simulink model "rocky_motor_disturb"  (R2022a)
settings: Solver=VariableStepAuto  StartTime=0.0  StopTime=2  RelTol=1e-3
model workspace (MAT data in the model file):
  m = 1000
values from neighbouring files (symbols this model uses):
  ci = 1    [rocky_constants.m]
  g = 9.81    [Rocky_closed_loop_poles.m]    (also in Rocky_closed_loop_poles_again.m; Rocky_closed_loop_poles_fresh_file.m; polederivation_CA.m; rocky_constants.m = 9.8)
  ji = 10    [rocky_constants.m]
  jp = 20    [rocky_constants.m]
  ki = 1.9509e+03    (= 1950.9)    [rocky_constants.m]
  kmotor = .92    (= 0.92)    [rocky_constants.m]
  kp = 2.2104e+03    (= 2210.4)    [rocky_constants.m]
  l = 0.4529    [Rocky_closed_loop_poles.m]    (also in Rocky_closed_loop_poles_again.m = 0.5588; Rocky_closed_loop_poles_fresh_file.m = 0.5588; polederivation_CA.m = 0.45; rocky_constants.m = 0.4)
  tau = .0511    (= 0.0511)    [rocky_constants.m]
settings Model: Creator=clee1  LastModifiedBy=ayydin
settings SolverCC: AlgebraicLoopSolver=TrustRegion
settings DebuggingCC: UnconnectedInputMsg=warning  UnconnectedOutputMsg=warning  UnconnectedLineMsg=warning  SFMachineParentedDataDiag=warning

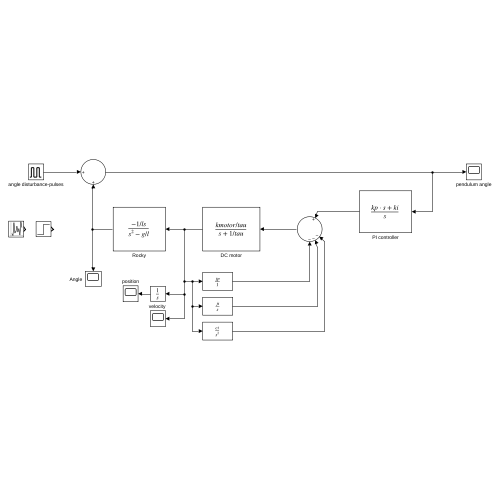
[thumbnail: Simulink's stored preview of the top-level diagram]
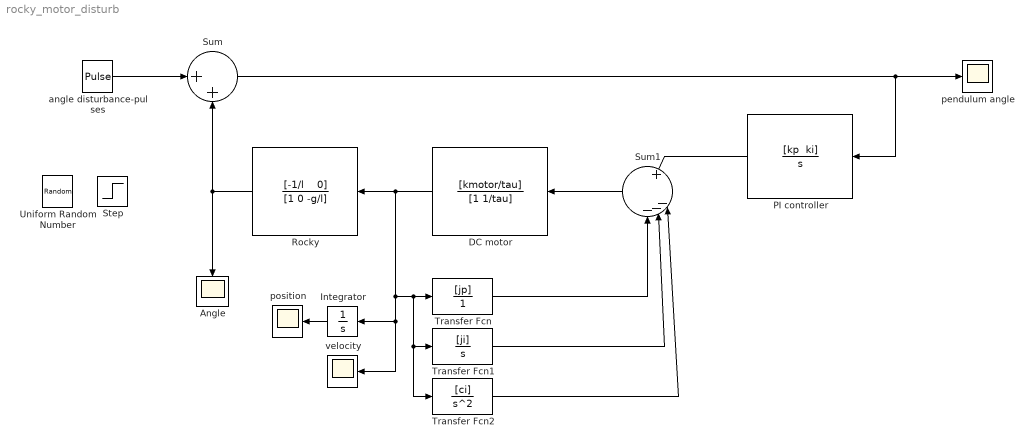
== system rocky_motor_disturb ==
  Angle : Scope
  DC motor : TransferFcn  Numerator=[kmotor/tau]  Denominator=[1 1/tau]
  Integrator : Integrator
  PI controller : TransferFcn  Numerator="[kp  ki]"  Denominator=[1 0 ]
  Rocky : TransferFcn  Numerator="[-1/l    0]"  Denominator=[1 0 -g/l]
  Step : Step  After=.1  SampleTime=0
  Sum : Sum  Inputs=|++
  Sum1 : Sum  Inputs=|+|||---
  Transfer Fcn : TransferFcn  Numerator=[jp]  Denominator=[1]
  Transfer Fcn1 : TransferFcn  Numerator=[ji]  Denominator=[1 0]
  Transfer Fcn2 : TransferFcn  Numerator=[ci]  Denominator=[1 0 0]
  Uniform Random Number : UniformRandomNumber  SampleTime=20
  angle disturbance-pulses : DiscretePulseGenerator  PulseType=Time based  Amplitude=.1  Period=10  PulseWidth=.1  PhaseDelay=.5
  pendulum angle : Scope
  position : Scope
  "velocity " : Scope
  wires:
  Rocky/1 -> Sum/2, Angle/1
  Sum/1 -> PI controller/1, pendulum angle/1
  angle disturbance-pulses/1 -> Sum/1
  DC motor/1 -> Transfer Fcn2/1, Transfer Fcn1/1, Transfer Fcn/1, "velocity "/1, Integrator/1, Rocky/1
  Integrator/1 -> position/1
  PI controller/1 -> Sum1/1
  Sum1/1 -> DC motor/1
  Transfer Fcn/1 -> Sum1/4
  Transfer Fcn1/1 -> Sum1/3
  Transfer Fcn2/1 -> Sum1/2
